simulink model "HoppingLEGV2_brisi"  (Simulink 7.7)
settings: Solver=ode3  StartTime=0.0  StopTime=5  FixedStep=Td  RelTol=1e-3
values from neighbouring files (symbols this model uses):
  Td = pi/wd    [AnalizaOscilatora.m]    (also in Start.m = 0.001)
libraries: vrlib x1
settings Model: Creator=Alan Mutka  LastModifiedBy=Alan Mutka

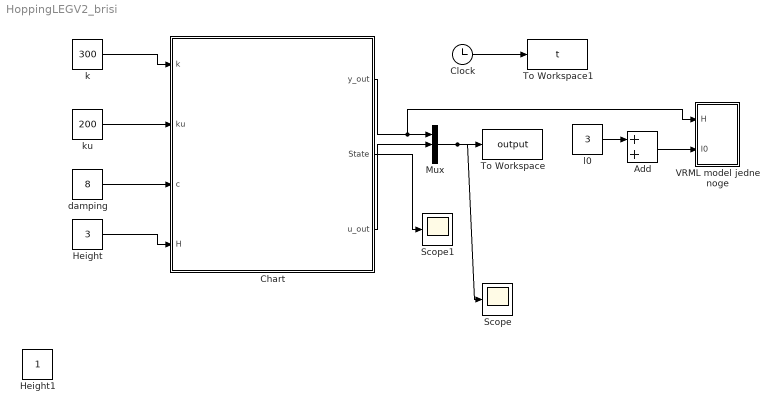
== system HoppingLEGV2_brisi ==
  Add : Sum
  Chart : Stateflow chart  TreatAsAtomicUnit=on
  Clock : Clock
      settings: Decimation=10
  Height : Constant  Value=3
  Height1 : Constant
  Mux : Mux  Inputs=3
  Scope : Scope
      settings: TimeRange=3  YMin=0  YMax=6.5
  Scope1 : Scope
      settings: TimeRange=3  YMin=1  YMax=1
  To Workspace : ToWorkspace  VariableName=output  SampleTime=Td  SaveFormat=Array
  To Workspace1 : ToWorkspace  VariableName=t  SampleTime=Td  SaveFormat=Array
  VRML model jedne noge : Subsystem
  damping : Constant  Value=8
  k : Constant  Value=300
  ku : Constant  Value=200
  l0 : Constant  Value=3
  wires:
  Chart/1(y_out) -> Mux/1, VRML model jedne noge/1(H)
  Mux/1 -> Scope/1, To Workspace/1
  Clock/1 -> To Workspace1/1
  damping/1 -> Chart/3(c)
  k/1 -> Chart/1(k)
  Height/1 -> Chart/4(H)
  l0/1 -> Add/1
  Add/1 -> VRML model jedne noge/2(I0)
  Chart/3(u_out) -> Mux/2
  Chart/2(State) -> Scope1/1
  ku/1 -> Chart/2(ku)

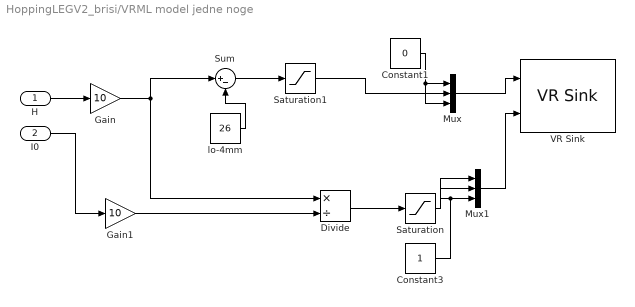
== system HoppingLEGV2_brisi/VRML model jedne noge ==
  H : Inport
  I0 : Inport  Port=2
  Constant1 : Constant  Value=0
  Constant3 : Constant
  Divide : Product  Inputs=*/
  Gain : Gain  Gain=10
  Gain1 : Gain  Gain=10
  Mux : Mux  Inputs=3
  Mux1 : Mux  Inputs=3
  Saturation : Saturate  UpperLimit=1  LowerLimit=0.5
  Saturation1 : Saturate  UpperLimit=10000  LowerLimit=4
  Sum : Sum  Inputs=|+-
  VR Sink : vrlib/VR Sink  SampleTime=-1  ViewEnable=on  RemoteChange=off  RemoteView=on  FieldsWritten=ALFA.translation.3.1.1.double#Opruga.scale.3.1.1.double  WorldFileName=B:\LARICS_GIT\LARICS-flying-Robin\@_LEG\VRML_MODEL\skakac.WRL  AutoView=off  VideoDimensions=[]  FigureProperties={}
  lo-4mm : Constant  Value=26
  wires:
  I0/1 -> Gain1/1
  H/1 -> Gain/1
  Sum/1 -> Saturation1/1
  lo-4mm/1 -> Sum/2
  Divide/1 -> Saturation/1
  Saturation1/1 -> Mux/2
  Constant3/1 -> Mux1/3, Mux1/1
  Saturation/1 -> Mux1/2
  Mux1/1 -> VR Sink/2
  Mux/1 -> VR Sink/1
  Constant1/1 -> Mux/3, Mux/1
  Gain/1 -> Divide/1, Sum/1
  Gain1/1 -> Divide/2

== stateflow chart Chart ==
  settings: updateMethod=CONTINUOUS
  state Swing
    du:
    y_dot=yv;
    yv_dot=-u*(k/m1+ku/m1)-uv*c/m1-g+k*l0/m1-k*s0/m1+ku*u0/m1;
    u_dot=uv;
    uv_dot=-u*(k/m1+ku/m1+k/m2+ku/m2)-uv*(c/m1+c/m2)+k*l0/m1+k*l0/m2-k*s0/m1-k*s0/m2+ku*u0/m1+ku*u0/m2;
    //output
    y_out = y;
    u_out=y-u;
    State=l0-u;
  state Stancedown
    du:
    y_dot = yv;
    yv_dot = ku/m1*(u0-u) -g;
    u_dot=uv;
    uv_dot=k/m2*y+yv*c/m2-u*(ku/m1+k/m2+ku/m2)-uv*c/m2 -k*s0/m2+ku*u0/m1+ku*u0/m2;
    y_out = y;
    u_out=y-u;
    State = y-u;
  (default) -> Swing : {
      | y=H;yv=0;
      | u=1;uv=0;
      | }
  Swing -> Stancedown : [y<=l0 && yv<0]
      | {
      |
      |
      |
      | }
  Stancedown -> Swing : [y>l0 && yv>0]
      | {
      |
      |
      |
      | }
  data: yv local double; y_out output double; y local double; k input double =800; ku input double =10000; m1 constant double =0.1; l0 constant double =2; c input double =6; H input double; State output double; u local double; uv local double; m2 constant double =0.01; u_out output double; s0 constant double =1; g constant double =9.81; u0 constant double =1
  data yv settings: updateMethod=SF_CONTINUOUS_TIME_DATA
  data y settings: updateMethod=SF_CONTINUOUS_TIME_DATA
  data H settings: updateMethod=SF_CONTINUOUS_TIME_DATA
  data u settings: updateMethod=SF_CONTINUOUS_TIME_DATA
  data uv settings: updateMethod=SF_CONTINUOUS_TIME_DATA
